simulink model "Microgrid_ITM_client"  (R2025b)
settings: Solver=FixedStepAuto  StartTime=0.0  StopTime=0.05  FixedStep=5e-7  RelTol=1e-3
InitFcn:
  | clear;
  | setup_two_pc_cosim();
  | clear Server_co_TLM Client_co_TLM
  | rehash;
  | release_two_pc_tcp_ports();
  | Vline = 380;%Rated RMS of Line Voltage
  | Vdc = 750;%DC voltage
  | Vac = sqrt(2)*Vline/sqrt(3);%Amplitude of Phase to Neutral Volatge
  | P = 10*10^(3);%Rate Power
  | f=50;%Rated Frequency
  | Wb=2*pi*f;%Rated Angular Frequency
  | fsw1=10e3;  %INV1 switching frequency
  | 
  | %Base Value of PU System
  | Vp=Vac;%Voltage
  | Ip=2/3*P/Vp;%Current
  | Zb = Vp/Ip;%Impedance
  | Lb=Zb/2/pi/f;%Inductance
  | Cb=1/(2*pi*f*Zb);%Capacitance
  | 
  | %Network Parameters
  | R1_pu=0.1/Zb;R1=R1_pu*Zb;
  | R2_pu=0.1/Zb;R2=R2_pu*Zb;
  | R3_pu=0.1/Zb;R3=R3_pu*Zb;
  | R4_pu=0.1/Zb;R4=R4_pu*Zb;
  | L1_pu=2e-3/Lb;L1=L1_pu*Lb;
  | L2_pu=2e-3/Lb;L2=L2_pu*Lb;
  | L3_pu=2e-3/Lb;L3=L3_pu*Lb;
  | L4_pu=2e-3/Lb;L4=L4_pu*Lb;
  | 
  | %Load Parameters
  | Rload1_pu=Vp/Ip/Zb;Rload1=Rload1_pu*Zb;
  | Rload2_pu=Vp/Ip/Zb;Rload2=Rload2_pu*Zb;
  | Rload3_pu=Vp/Ip/Zb;Rload3=Rload3_pu*Zb;
  | 
  | %Virtual Impedance
  | Rv_pu=0.05;
  | Xv_pu=0.2;
  | 
  | Lc=2.5e-3;
StopFcn:
  | %% StopFcn: save ITM client-side results
  | 
  | % 获取模型所在目录
  | modelName = bdroot;
  | modelFile = get_param(modelName, 'FileName');
  | 
  | if isempty(modelFile)
  |     % 模型还没有保存时，使用当前工作目录
  |     modelDir = pwd;
  | else
  |     modelDir = fileparts(modelFile);
  | end
  | 
  | % 定义并创建 result 文件夹
  | resultDir = fullfile(modelDir, 'result');
  | 
  | if ~exist(resultDir, 'dir')
  |     mkdir(resultDir);
  | end
  | 
  | % 需要保存的 Client-side 工作区变量
  | variableNames = {
  |     'client_voltage'
  |     'client_current'
  |     'client_PQ'
  |     'client_omega'
  | };
  | 
  | clientITMData = struct();
  | 
  | for k = 1:numel(variableNames)
  | 
  |     originalName = variableNames{k};
  |     saveName = [originalName, '_client_ITM'];
  | 
  |     variableExists = evalin( ...
  |         'base', ...
  |         sprintf('exist(''%s'', ''var'')', originalName));
  | 
  |     if variableExists
  |         clientITMData.(saveName) = evalin('base', originalName);
  |     else
  |         warning( ...
  |             'StopFcn:MissingVariable', ...
  |             'Variable "%s" was not found in the base workspace.', ...
  |             originalName);
  |     end
  | end
  | 
  | % 保存文件
  | saveFile = fullfile(resultDir, 'client_ITM.mat');
  | save(saveFile, '-struct', 'clientITMData');
  | 
  | fprintf('ITM client-side results saved to:\n%s\n', saveFile);
undefined symbols (not defined in the file or in its folder): DiscIntNeverNeededParam
libraries: spsThreePhaseSeriesRLCBranchLib x4, spsControlledCurrentSourceLib x3, spsControlledVoltageSourceLib x3, slpidlib x3, spsabctodq0Lib x3, spsThreePhaseVIMeasurementLib x3, spsThreePhaseTransformerTwoWindingsLib x2, spsDCVoltageSourceLib x1, spsGroundLib x1, spsPWMGenerator2LevelLib x1, spsPower3phInstantaneousLib x1, spsdq0toabcLib x1
settings Model: Creator=L  LastModifiedBy=Yuming
settings SolverCC: AlgebraicLoopSolver=TrustRegion
settings DataIOCC: LimitDataPoints=on  SaveFormat=Array  ReturnWorkspaceOutputs=off
settings OptimizationCC: ReuseModelBlockBuffer=off  LifeSpan=inf
settings DebuggingCC: UnderspecifiedInitializationDetection=Classic  MergeDetectMultiDrivingBlocksExec=none  SolverPrmCheckMsg=warning  UnconnectedInputMsg=warning  UnconnectedOutputMsg=warning  UnconnectedLineMsg=warning  StateNameClashWarn=warning  SFUnexpectedBacktrackingDiag=warning  SFNoUnconditionalDefaultTransitionDiag=warning  SFExecutionAtInitializationDiag=none  ArithmeticOperatorsInVariantConditions=warning
settings HardwareCC: ProdBitPerPointer=32.0  ProdBitPerSizeT=32.0  ProdBitPerPtrDiffT=32.0  ProdLargestAtomicFloat=None  ProdIntDivRoundTo=Undefined  ProdEndianess=Unspecified  ProdWordSize=32.0  ProdHWDeviceType=32-bit Generic
settings ModelReferenceCC: EnableRefExpFcnMdlSchedulingChecks=on  PropagateSignalLabelsOutOfModel=off
settings SFSimCC: SimUseLocalCustomCode=off  CustomCodeUndefinedFunction=UseInterfaceOnly
settings RTWCC: RTWUseLocalCustomCode=off  GPUComputeCapability=3.5  DLArmComputeVersion=19.05
settings CodeAppCC: StateflowObjectComments=on
settings GRTTargetCC: TargetLangStandard=C89/C90 (ANSI)
settings ConfigComp: CovMetricSettings=dw  CovSaveCumulativeToWorkspaceVar=on  CovSaveSingleToWorkspaceVar=on  CovExternalEMLEnable=off
settings SimscapeCC: SimscapeNormalizeSystem=off

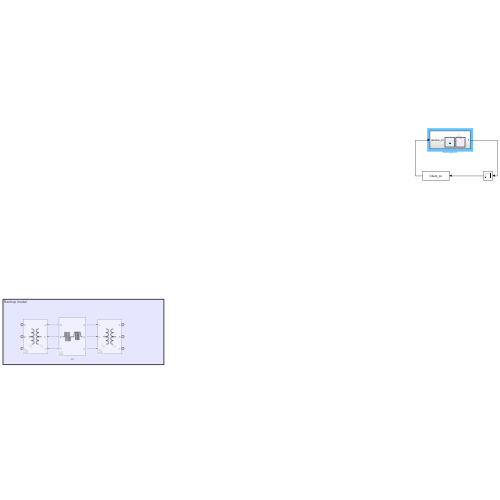
[thumbnail: Simulink's stored preview of the top-level diagram]
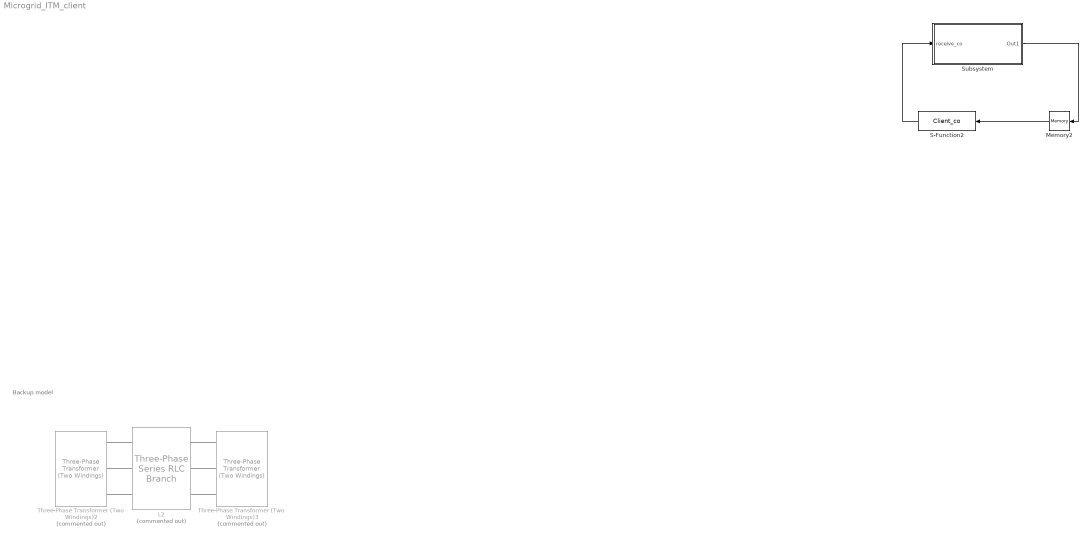
== system Microgrid_ITM_client ==
  note: Backup model
  L2 : spsThreePhaseSeriesRLCBranchLib/Three-Phase Series RLC Branch  Commented=on  LConnTagsString=A|B|C  RConnTagsString=A|B|C  BranchType=RL  Resistance=R2  Inductance=L2  Capacitance=1e-6  Measurements=None
  Memory2 : Memory
  S-Function2 : S-Function  FunctionName=Client_co  SFunctionDeploymentMode=off  EnableBusSupport=off
  Subsystem : Subsystem
  Three-Phase Transformer (Two Windings)2 : spsThreePhaseTransformerTwoWindingsLib/Three-Phase Transformer (Two Windings)  Commented=on  Winding1Connection=Yg  Winding2Connection=Yg  CoreType=Three single-phase transformers  SetSaturation=off  Hysteresis=off  DataFile='hysteresis'  SetInitialFlux=off  Measurements=None  UNITS=pu  NominalPower=[ 250e6 , 50 ]  Winding1=[ 380e3 , 0.002 , 0.08 ]  Winding2=[ 33e3 , 0.002 , 0.08 ]  Rm=500  Lm=500  L0=0.5  Saturation=[ 0,0 ; 0.0024,1.2 ; 1.0,1.52 ]  InitialFluxes=[ 0.8 , -0.8 , 0.7 ]  BreakLoop=off  DiscreteSolver=Trapezoidal iterative  DataType=off  TransfoNumber=1
  Three-Phase Transformer (Two Windings)3 : spsThreePhaseTransformerTwoWindingsLib/Three-Phase Transformer (Two Windings)  Commented=on  Winding1Connection=Yg  Winding2Connection=Yg  CoreType=Three single-phase transformers  SetSaturation=off  Hysteresis=off  DataFile='hysteresis'  SetInitialFlux=off  Measurements=None  UNITS=pu  NominalPower=[ 250e6 , 50 ]  Winding1=[ 33e3 , 0.002 , 0.08 ]  Winding2=[ 380 , 0.002 , 0.08 ]  Rm=500  Lm=500  L0=0.5  Saturation=[ 0,0 ; 0.0024,1.2 ; 1.0,1.52 ]  InitialFluxes=[ 0.8 , -0.8 , 0.7 ]  BreakLoop=off  DiscreteSolver=Trapezoidal iterative  DataType=off  TransfoNumber=1
  wires:
  Memory2/1 -> S-Function2/1
  S-Function2/1 -> Subsystem/1(receive_co)
  Subsystem/1(Out1) -> Memory2/1
  connections:
  Three-Phase Transformer (Two Windings)3/RConn1 -- L2/RConn1
  Three-Phase Transformer (Two Windings)3/RConn2 -- L2/RConn2
  Three-Phase Transformer (Two Windings)3/RConn3 -- L2/RConn3
  Three-Phase Transformer (Two Windings)2/RConn1 -- L2/LConn1
  Three-Phase Transformer (Two Windings)2/RConn2 -- L2/LConn2
  Three-Phase Transformer (Two Windings)2/RConn3 -- L2/LConn3

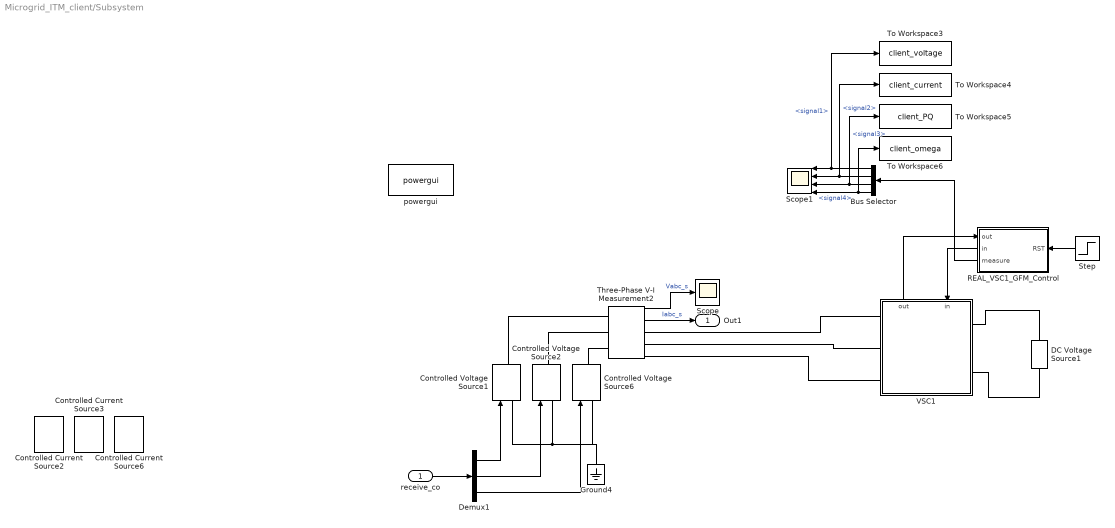
== system Microgrid_ITM_client/Subsystem ==
  receive_co : Inport
  Bus Selector : BusSelector  OutputSignals=signal1,signal2,signal3,signal4
  Controlled Current Source2 : spsControlledCurrentSourceLib/Controlled Current Source  Initialize=on  Source_Type=AC  Amplitude=0  Phase=0  Frequency=0  Measurements=None
  Controlled Current Source3 : spsControlledCurrentSourceLib/Controlled Current Source  Initialize=on  Source_Type=AC  Amplitude=0  Phase=0  Frequency=0  Measurements=None
  Controlled Current Source6 : spsControlledCurrentSourceLib/Controlled Current Source  Initialize=on  Source_Type=AC  Amplitude=0  Phase=0  Frequency=0  Measurements=None
  Controlled Voltage Source1 : spsControlledVoltageSourceLib/Controlled Voltage Source  Initialize=on  Source_Type=AC  Amplitude=0  Phase=0  Frequency=0  Measurements=None
  Controlled Voltage Source2 : spsControlledVoltageSourceLib/Controlled Voltage Source  Initialize=on  Source_Type=AC  Amplitude=0  Phase=0  Frequency=0  Measurements=None
  Controlled Voltage Source6 : spsControlledVoltageSourceLib/Controlled Voltage Source  Initialize=on  Source_Type=AC  Amplitude=0  Phase=0  Frequency=0  Measurements=None
  DC Voltage Source1 : spsDCVoltageSourceLib/DC Voltage Source  Amplitude=Vdc  Measurements=None
  Demux1 : Demux  Outputs=3
  Ground4 : spsGroundLib/Ground  LConnTagsString=a
  REAL_VSC1_GFM_Control : Subsystem
      settings: PortSchema="{\"entries\":[{\"content\":{\"sides\":[{\"content\":{\"connectorIds\":[\"In1\"]},\"type\":\"ConnectorPlacement.EquallySpacedRectSide\",\"uuid\":\"8a24280a-bafa-4af5-a0f6-406aa9a59b4a\"},{\"content\":{\"connectorIds\":[\"In2\",\"Out1\",\"Out2\"],\"side\":\"RIGHT\"},\"type\":\"ConnectorPlacement.EquallySpacedRectSide\",\"uuid\":\"7d4db3bb-9035-4630-ac97-c56e5fe5f777\"},{\"content\":{\"side\":\"TOP\"},\"type\":\"ConnectorPlacement.EquallySpacedRectSide\",\"uuid\":\"cf83f05c-de7f-4d84-9d8a-6900bb43b99f\"}]},\"type\":\"ConnectorPlacement.EquallySpacedConnector\",\"uuid\":\"3f42a8c1-e25b-4642-96cc-07219abe8890\"}],\"packageUris\":[\"http://schema.mathworks.com/mf0/Connector/R2020b\"],\"version\":\"1.0\"}"
  Scope : Scope
      settings: ActiveDisplayYMinimum=-5.8273159155410254E+163  ActiveDisplayYMaximum=5.8951340842267878E+163  DataLoggingVariableName=ScopeData5
  Scope1 : Scope  NumInputPorts=4
      settings: ActiveDisplayYMinimum=-417.44619371330521  ActiveDisplayYMaximum=395.41957020213545  DataLoggingVariableName=ScopeData4
  Step : Step  Time=0.2  SampleTime=0
  Three-Phase V-I Measurement2 : spsThreePhaseVIMeasurementLib/Three-Phase V-I Measurement  VoltageMeasurement=phase-to-ground  SetLabelV=off  LabelV=Vabc_s  Vpu=off  VpuLL=off  CurrentMeasurement=yes  SetLabelI=off  LabelI=Iabc_s  Ipu=off  Pbase=100e6  Vbase=500e3  OutputType=Complex  PhasorSimulation=off  PSBequivalent=0
  To Workspace3 : ToWorkspace  VariableName=client_voltage  SaveFormat=Timeseries  SampleTime=-1
  To Workspace4 : ToWorkspace  VariableName=client_current  SaveFormat=Timeseries  SampleTime=-1
  To Workspace5 : ToWorkspace  VariableName=client_PQ  SaveFormat=Timeseries  SampleTime=-1
  To Workspace6 : ToWorkspace  VariableName=client_omega  SaveFormat=Timeseries  SampleTime=-1
  VSC1 : Subsystem
      settings: PortSchema="{\"entries\":[{\"content\":{\"sides\":[{\"content\":{\"connectorIds\":[\"LConn1\",\"LConn2\"]},\"type\":\"ConnectorPlacement.EquallySpacedRectSide\",\"uuid\":\"f9a47b7a-7ab9-4bc4-ba6a-b9374cb03391\"},{\"content\":{\"connectorIds\":[\"RConn1\",\"RConn2\",\"RConn3\"],\"side\":\"RIGHT\"},\"type\":\"ConnectorPlacement.EquallySpacedRectSide\",\"uuid\":\"cfb0475f-9637-449c-a598-06e77c9a1f18\"},{\"content\":{\"connectorIds\":[\"In1\",\"Out1\"],\"side\":\"TOP\"},\"type\":\"ConnectorPlacement.EquallySpacedRectSide\",\"uuid\":\"93622264-4e82-4ec9-8ad8-ec19c934a5ef\"},{\"content\":{\"side\":\"HIDDEN\"},\"type\":\"ConnectorPlacement.EquallySpacedRectSide\",\"uuid\":\"56686535-bc45-40fb-9bd4-cc49f520b447\"}]},\"type\":\"ConnectorPlacement.EquallySpacedConnector\",\"uuid\":\"6064451f-78f0-465c-b58b-22fa19e3979e\"}],\"packageUris\":[\"http://schema.mathworks.com/mf0/Connector/R2020b\"],\"version\":\"1.0\"}"
  powergui : spspowerguiLib/powergui  Priority=1  SimulationMode=Discrete  SampleTime=5e-7  frequency=60  Iterations=50  frequencyindice=0  Pbase=100e6  ErrMax=1e-4  UnitsV=kV  UnitsW=MW  buscounter=0  FunctionMessages=off  echomessages=off  EnableUseOfTLC=off  CurrentSourceSwitches=off  DisableSnubberDevices=off  DisableRonSwitches=off  DisableVfSwitches=off  DisplayEquations=off  AutomaticDiscreteSolvers=off  SolverType=Tustin/Backward Euler (TBE)  Interpol=off  ExternalGateDelay=off  methode=off  Ts=100  x0status=blocks  SPID=on  SwTol=0  HookPort=off  NonlinearTolerance=1e-4  nMaxIteration=100  ContinueOnMaxIteration=off  RestoreLinks=warning  ResistiveCurrentMeasurement=off  Frange=[0:2:500]  Ylog=off  Xlog=on  ShowGrid=off  save=off  variable=ZData  structure=0  ZoomFFT=off  StartTime=0.0  cycles=1  DisplayStyle=1  fundamental=60  FreqAxis=off  MaxFrequency=1000  frequencyindicesteady=1  RmsSteady=1  display=off
  Out1 : Outport
  wires:
  VSC1/1(out) -> REAL_VSC1_GFM_Control/2(out)
  Step/1 -> REAL_VSC1_GFM_Control/1(RST)
  REAL_VSC1_GFM_Control/1(in) -> VSC1/1(in)
  Demux1/2 -> Controlled Voltage Source2/1
  Demux1/3 -> Controlled Voltage Source6/1
  receive_co/1 -> Demux1/1
  Demux1/1 -> Controlled Voltage Source1/1
  REAL_VSC1_GFM_Control/2(measure) -> Bus Selector/1
  Bus Selector/1 -> To Workspace3/1, Scope1/1  "<signal1>"
  Bus Selector/3 -> To Workspace5/1, Scope1/3  "<signal3>"
  Bus Selector/4 -> To Workspace6/1, Scope1/4  "<signal4>"
  Bus Selector/2 -> To Workspace4/1, Scope1/2  "<signal2>"
  Three-Phase V-I Measurement2/1 -> Scope/1  "Vabc_s"
  Three-Phase V-I Measurement2/2 -> Out1/1  "Iabc_s"
  connections:
  DC Voltage Source1/RConn1 -- VSC1/LConn1
  VSC1/LConn2 -- DC Voltage Source1/LConn1
  Controlled Voltage Source1/RConn1 -- Three-Phase V-I Measurement2/LConn1
  Ground4/LConn1 -- Controlled Voltage Source6/LConn1 -- Controlled Voltage Source1/LConn1 -- Controlled Voltage Source2/LConn1
  Controlled Voltage Source2/RConn1 -- Three-Phase V-I Measurement2/LConn2
  Controlled Voltage Source6/RConn1 -- Three-Phase V-I Measurement2/LConn3
  Three-Phase V-I Measurement2/RConn1 -- VSC1/RConn1
  Three-Phase V-I Measurement2/RConn2 -- VSC1/RConn2
  Three-Phase V-I Measurement2/RConn3 -- VSC1/RConn3

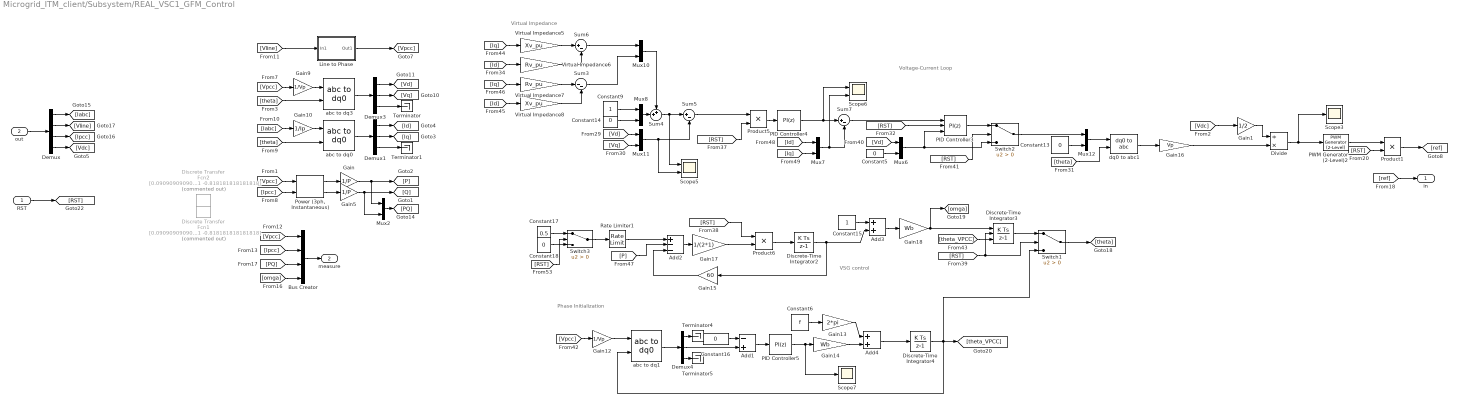
== system Microgrid_ITM_client/Subsystem/REAL_VSC1_GFM_Control ==
  note: Voltage-Current Loop
  note: VSG control
  note: Virtual Impedance
  note: Phase Initialization
  RST : Inport
  out : Inport  Port=2
  Add1 : Sum  Inputs=-+
  Add2 : Sum  Inputs=+--
  Add3 : Sum
  Add4 : Sum
  Bus Creator : BusCreator  Inputs=4
  Constant{5,13..14,16} (4 alike) : Constant  Value=0
  Constant15 : Constant
  Constant17 : Constant  Value=0.5  SampleTime=-1
  Constant18 : Constant  Value=0  SampleTime=-1
  Constant6 : Constant  Value=f
  Constant9 : Constant  SampleTime=-1
  Demux : Demux
  Demux1 : Demux  Outputs=3
  Demux3 : Demux  Outputs=3
  Demux4 : Demux  Outputs=3
  Discrete Transfer Fcn1 : DiscreteTransferFcn  Commented=on  Numerator=[0.090909090909091 0.090909090909091]  Denominator=[1 -0.818181818181818]
  Discrete Transfer Fcn2 : DiscreteTransferFcn  Commented=on  Numerator=[0.090909090909091 0.090909090909091]  Denominator=[1 -0.818181818181818]
  Discrete-Time Integrator2 : DiscreteIntegrator  SampleTime=1/fsw1  ICPrevOutput=DiscIntNeverNeededParam  ICPrevScaledInput=DiscIntNeverNeededParam
  Discrete-Time Integrator3 : DiscreteIntegrator  ExternalReset=rising  InitialConditionSource=external  SampleTime=1/fsw1  ICPrevOutput=DiscIntNeverNeededParam  ICPrevScaledInput=DiscIntNeverNeededParam
  Discrete-Time Integrator4 : DiscreteIntegrator  SampleTime=1/fsw1  ICPrevOutput=DiscIntNeverNeededParam  ICPrevScaledInput=DiscIntNeverNeededParam
  Divide : Product  Inputs=/*
  Gain : Gain  Gain=1/P
  Gain1 : Gain  Gain=1/2
  Gain10 : Gain  Gain=1/Ip
  Gain12 : Gain  Gain=1/Vp
  Gain13 : Gain  Gain=2*pi
  Gain14 : Gain  Gain=Wb
  Gain15 : Gain  Gain=60
  Gain16 : Gain  Gain=Vp
  Gain17 : Gain  Gain=1/(2*1)
  Gain18 : Gain  Gain=Wb
  Gain5 : Gain  Gain=1/P
  Gain9 : Gain  Gain=1/Vp
  Line to Phase : Subsystem
  Mux{2,6..8,10..12} (7 alike) : Mux  Inputs=2
  PID Controller3 : slpidlib/PID Controller  Controller=PI  Form=Parallel  TimeDomain=Discrete-time  UseExternalTs=off  SampleTime=1/fsw1  IntegratorMethod=Forward Euler  FilterMethod=Forward Euler  ControllerParametersSource=internal  P=0.5  I=100  UseKiTs=off  D=0  UseExternalDerivativeSource=off  N=100  UseFilter=on  TunerSelectOption=Transfer Function Based (PID Tuner App)  InitialConditionSource=external  InitialConditionForIntegrator=0  InitialConditionForFilter=0  DifferentiatorICPrevScaledInput=0  ExternalReset=rising  TrackingMode=off  Kt=1  LimitOutput=off  SatLimitsSource=internal  UpperSaturationLimit=inf  LowerSaturationLimit=-inf  LinearizeAsGain=on  AntiWindupMode=none  Kb=1  LimitIntegrator=off  UpperIntegratorSaturationLimit=inf  LowerIntegratorSaturationLimit=-inf  POutMin=[]  POutMax=[]  IOutMin=[]  IOutMax=[]  DOutMin=[]  DOutMax=[]  NOutMin=[]  NOutMax=[]  SumOutMin=[]  SumOutMax=[]  SaturationOutMin=[]  SaturationOutMax=[]  PParamMin=[]  PParamMax=[]  IParamMin=[]  IParamMax=[]  DParamMin=[]  DParamMax=[]  NParamMin=[]  NParamMax=[]  KbParamMin=[]  KbParamMax=[]  KtParamMin=[]  KtParamMax=[]  KbOutMin=[]  KbOutMax=[]  KtOutMin=[]  KtOutMax=[]  IntegratorOutMin=[]  IntegratorOutMax=[]  FilterOutMin=[]  FilterOutMax=[]  SumI1OutMin=[]  SumI1OutMax=[]  SumI2OutMin=[]  SumI2OutMax=[]  SumI3OutMin=[]  SumI3OutMax=[]  SumI4OutMin=[]  SumI4OutMax=[]  SumDOutMin=[]  SumDOutMax=[]  DifferentiatorOutMin=[]  DifferentiatorOutMax=[]  FilterDiffOutCoefMin=[]  FilterDiffOutCoefMax=[]  ReciprocalOutMin=[]  ReciprocalOutMax=[]  SumDenOutMin=[]  SumDenOutMax=[]  SumNumOutMin=[]  SumNumOutMax=[]  DivideOutMin=[]  DivideOutMax=[]  UdiffTsProdOutMin=[]  UdiffTsProdOutMax=[]  NTsProdOutMin=[]  NTsProdOutMax=[]  UintegralTsProdOutMin=[]  UintegralTsProdOutMax=[]  UngainTsProdOutMin=[]  UngainTsProdOutMax=[]  ClampingZeroOutDataTypeStr=Inherit: Inherit via back propagation  ClampingZeroOutMin=[]  ClampingZeroOutMax=[]  FilterDenConstantOutDataTypeStr=Inherit: Inherit via back propagation  FilterDenConstantOutMin=[]  FilterDenConstantOutMax=[]  PCopyOutDataTypeStr=Inherit: Inherit via back propagation  PCopyOutMin=[]  PCopyOutMax=[]  NCopyOutDataTypeStr=Inherit: Inherit via back propagation  NCopyOutMin=[]  NCopyOutMax=[]  IntegratorContinuousStateAttributes=''  IntegratorStateMustResolveToSignalObject=off  IntegratorRTWStateStorageClass=Auto  FilterContinuousStateAttributes=''  FilterStateMustResolveToSignalObject=off  FilterRTWStateStorageClass=Auto  ParallelPVariant=InternalParameters  IdealPVariant=Disabled  IVariant=InternalParameters  DVariant=Disabled  IntegratorVariant=Discrete  SatVariant=Disabled  AWVariant=Passthrough  PCopyVariant=Disabled  TRVariant=Disabled  FdbkBlocksVariant=Forward  IdealPFdbkVariant=Disabled  SatFdbkVariant=Disabled  DerivativeFilterVariant=Disabled  NVariant=Disabled  NCopyVariant=Disabled_SignalSpec  FilterICVariant=Disabled  IntegratorICVariant=ExternalICs  ExternalResetVariant=ExternalReset  TRSumVariant=Passthrough  SumFdbkVariant=Disabled  SumVariant=Sum_PI  TsampFilterVariant=InternalTs  TsampNgainVariant=Passthrough  TsampIntegralVariant=Disabled_SignalSpec  ExternalSaturationOutDataTypeStr=Inherit: Same as second input  DerivativeSourceVariant=Disabled  PreIntVariant=InternalPreInt
  PID Controller4 : slpidlib/PID Controller  Controller=PI  Form=Parallel  TimeDomain=Discrete-time  UseExternalTs=off  SampleTime=1/fsw1  IntegratorMethod=Forward Euler  FilterMethod=Forward Euler  ControllerParametersSource=internal  P=0.1  I=200  UseKiTs=off  D=0  UseExternalDerivativeSource=off  N=100  UseFilter=on  TunerSelectOption=Transfer Function Based (PID Tuner App)  InitialConditionSource=internal  InitialConditionForIntegrator=0  InitialConditionForFilter=0  DifferentiatorICPrevScaledInput=0  ExternalReset=none  TrackingMode=off  Kt=1  LimitOutput=off  SatLimitsSource=internal  UpperSaturationLimit=inf  LowerSaturationLimit=-inf  LinearizeAsGain=on  AntiWindupMode=none  Kb=1  LimitIntegrator=off  UpperIntegratorSaturationLimit=inf  LowerIntegratorSaturationLimit=-inf  POutMin=[]  POutMax=[]  IOutMin=[]  IOutMax=[]  DOutMin=[]  DOutMax=[]  NOutMin=[]  NOutMax=[]  SumOutMin=[]  SumOutMax=[]  SaturationOutMin=[]  SaturationOutMax=[]  PParamMin=[]  PParamMax=[]  IParamMin=[]  IParamMax=[]  DParamMin=[]  DParamMax=[]  NParamMin=[]  NParamMax=[]  KbParamMin=[]  KbParamMax=[]  KtParamMin=[]  KtParamMax=[]  KbOutMin=[]  KbOutMax=[]  KtOutMin=[]  KtOutMax=[]  IntegratorOutMin=[]  IntegratorOutMax=[]  FilterOutMin=[]  FilterOutMax=[]  SumI1OutMin=[]  SumI1OutMax=[]  SumI2OutMin=[]  SumI2OutMax=[]  SumI3OutMin=[]  SumI3OutMax=[]  SumI4OutMin=[]  SumI4OutMax=[]  SumDOutMin=[]  SumDOutMax=[]  DifferentiatorOutMin=[]  DifferentiatorOutMax=[]  FilterDiffOutCoefMin=[]  FilterDiffOutCoefMax=[]  ReciprocalOutMin=[]  ReciprocalOutMax=[]  SumDenOutMin=[]  SumDenOutMax=[]  SumNumOutMin=[]  SumNumOutMax=[]  DivideOutMin=[]  DivideOutMax=[]  UdiffTsProdOutMin=[]  UdiffTsProdOutMax=[]  NTsProdOutMin=[]  NTsProdOutMax=[]  UintegralTsProdOutMin=[]  UintegralTsProdOutMax=[]  UngainTsProdOutMin=[]  UngainTsProdOutMax=[]  ClampingZeroOutDataTypeStr=Inherit: Inherit via back propagation  ClampingZeroOutMin=[]  ClampingZeroOutMax=[]  FilterDenConstantOutDataTypeStr=Inherit: Inherit via back propagation  FilterDenConstantOutMin=[]  FilterDenConstantOutMax=[]  PCopyOutDataTypeStr=Inherit: Inherit via back propagation  PCopyOutMin=[]  PCopyOutMax=[]  NCopyOutDataTypeStr=Inherit: Inherit via back propagation  NCopyOutMin=[]  NCopyOutMax=[]  IntegratorContinuousStateAttributes=''  IntegratorStateMustResolveToSignalObject=off  IntegratorRTWStateStorageClass=Auto  FilterContinuousStateAttributes=''  FilterStateMustResolveToSignalObject=off  FilterRTWStateStorageClass=Auto  ParallelPVariant=InternalParameters  IdealPVariant=Disabled  IVariant=InternalParameters  DVariant=Disabled  IntegratorVariant=Discrete  SatVariant=Disabled  AWVariant=Passthrough  PCopyVariant=Disabled  TRVariant=Disabled  FdbkBlocksVariant=Forward  IdealPFdbkVariant=Disabled  SatFdbkVariant=Disabled  DerivativeFilterVariant=Disabled  NVariant=Disabled  NCopyVariant=Disabled_SignalSpec  FilterICVariant=Disabled  IntegratorICVariant=InternalICs  ExternalResetVariant=Disabled  TRSumVariant=Passthrough  SumFdbkVariant=Disabled  SumVariant=Sum_PI  TsampFilterVariant=InternalTs  TsampNgainVariant=Passthrough  TsampIntegralVariant=Disabled_SignalSpec  ExternalSaturationOutDataTypeStr=Inherit: Same as second input  DerivativeSourceVariant=Disabled  PreIntVariant=InternalPreInt
  PID Controller5 : slpidlib/PID Controller  Controller=PI  Form=Parallel  TimeDomain=Discrete-time  UseExternalTs=off  SampleTime=1/fsw1  IntegratorMethod=Forward Euler  FilterMethod=Forward Euler  ControllerParametersSource=internal  P=2  I=5  UseKiTs=off  D=0  UseExternalDerivativeSource=off  N=100  UseFilter=on  TunerSelectOption=Transfer Function Based (PID Tuner App)  InitialConditionSource=internal  InitialConditionForIntegrator=0  InitialConditionForFilter=0  DifferentiatorICPrevScaledInput=0  ExternalReset=none  TrackingMode=off  Kt=1  LimitOutput=off  SatLimitsSource=internal  UpperSaturationLimit=inf  LowerSaturationLimit=-inf  LinearizeAsGain=on  AntiWindupMode=none  Kb=1  LimitIntegrator=off  UpperIntegratorSaturationLimit=inf  LowerIntegratorSaturationLimit=-inf  POutMin=[]  POutMax=[]  IOutMin=[]  IOutMax=[]  DOutMin=[]  DOutMax=[]  NOutMin=[]  NOutMax=[]  SumOutMin=[]  SumOutMax=[]  SaturationOutMin=[]  SaturationOutMax=[]  PParamMin=[]  PParamMax=[]  IParamMin=[]  IParamMax=[]  DParamMin=[]  DParamMax=[]  NParamMin=[]  NParamMax=[]  KbParamMin=[]  KbParamMax=[]  KtParamMin=[]  KtParamMax=[]  KbOutMin=[]  KbOutMax=[]  KtOutMin=[]  KtOutMax=[]  IntegratorOutMin=[]  IntegratorOutMax=[]  FilterOutMin=[]  FilterOutMax=[]  SumI1OutMin=[]  SumI1OutMax=[]  SumI2OutMin=[]  SumI2OutMax=[]  SumI3OutMin=[]  SumI3OutMax=[]  SumI4OutMin=[]  SumI4OutMax=[]  SumDOutMin=[]  SumDOutMax=[]  DifferentiatorOutMin=[]  DifferentiatorOutMax=[]  FilterDiffOutCoefMin=[]  FilterDiffOutCoefMax=[]  ReciprocalOutMin=[]  ReciprocalOutMax=[]  SumDenOutMin=[]  SumDenOutMax=[]  SumNumOutMin=[]  SumNumOutMax=[]  DivideOutMin=[]  DivideOutMax=[]  UdiffTsProdOutMin=[]  UdiffTsProdOutMax=[]  NTsProdOutMin=[]  NTsProdOutMax=[]  UintegralTsProdOutMin=[]  UintegralTsProdOutMax=[]  UngainTsProdOutMin=[]  UngainTsProdOutMax=[]  ClampingZeroOutDataTypeStr=Inherit: Inherit via back propagation  ClampingZeroOutMin=[]  ClampingZeroOutMax=[]  FilterDenConstantOutDataTypeStr=Inherit: Inherit via back propagation  FilterDenConstantOutMin=[]  FilterDenConstantOutMax=[]  PCopyOutDataTypeStr=Inherit: Inherit via back propagation  PCopyOutMin=[]  PCopyOutMax=[]  NCopyOutDataTypeStr=Inherit: Inherit via back propagation  NCopyOutMin=[]  NCopyOutMax=[]  IntegratorContinuousStateAttributes=''  IntegratorStateMustResolveToSignalObject=off  IntegratorRTWStateStorageClass=Auto  FilterContinuousStateAttributes=''  FilterStateMustResolveToSignalObject=off  FilterRTWStateStorageClass=Auto  ParallelPVariant=InternalParameters  IdealPVariant=Disabled  IVariant=InternalParameters  DVariant=Disabled  IntegratorVariant=Discrete  SatVariant=Disabled  AWVariant=Passthrough  PCopyVariant=Disabled  TRVariant=Disabled  FdbkBlocksVariant=Forward  IdealPFdbkVariant=Disabled  SatFdbkVariant=Disabled  DerivativeFilterVariant=Disabled  NVariant=Disabled  NCopyVariant=Disabled_SignalSpec  FilterICVariant=Disabled  IntegratorICVariant=InternalICs  ExternalResetVariant=Disabled  TRSumVariant=Passthrough  SumFdbkVariant=Disabled  SumVariant=Sum_PI  TsampFilterVariant=InternalTs  TsampNgainVariant=Passthrough  TsampIntegralVariant=Disabled_SignalSpec  ExternalSaturationOutDataTypeStr=Inherit: Same as second input  DerivativeSourceVariant=Disabled  PreIntVariant=InternalPreInt
  PWM Generator (2-Level)2 : spsPWMGenerator2LevelLib/PWM Generator (2-Level)  ModulatorType=Three-phase bridge (6 pulses)  ModulatorMode=Unsynchronized  Fc=fsw1  Pc=0  nF=27  MinMax="[ -1  1 ]"  SamplingTechnique=Asymmetrical regular (double edge)  ModulatingSignals=off  m=0.8  Freq=60  Phase=0  Ts=0  ShowCarrierOutport=off
  "Power (3ph, Instantaneous)" : spsPower3phInstantaneousLib/Power (3ph, Instantaneous)
  Product1 : Product
  Product5 : Product
  Product6 : Product
  Rate Limiter1 : RateLimiter  RisingSlewLimit=5  FallingSlewLimit=-5  SampleTimeMode=inherited
  Scope3 : Scope
      settings: ActiveDisplayYMinimum=-3.23588  ActiveDisplayYMaximum=3.22923
  Scope5 : Scope  NumInputPorts=2
      settings: ActiveDisplayYMinimum=-0.89875  ActiveDisplayYMaximum=1.61871
  Scope6 : Scope  NumInputPorts=2
      settings: ActiveDisplayYMinimum=-0.00056  ActiveDisplayYMaximum=0.00032  DataLoggingVariableName=ScopeData2
  Scope7 : Scope
      settings: ActiveDisplayYMinimum=-0.17841  ActiveDisplayYMaximum=0.07598  DataLoggingVariableName=ScopeData3
  Sum3 : Sum  Inputs=|--
  Sum4 : Sum  Inputs=++|
  Sum5 : Sum  Inputs=|+-
  Sum6 : Sum  Inputs=|+-
  Sum7 : Sum  Inputs=|+-
  Switch1 : Switch  Criteria=u2 > Threshold  SaturateOnIntegerOverflow=off  InputSameDT=off
  Switch2 : Switch  Criteria=u2 > Threshold  SaturateOnIntegerOverflow=off  InputSameDT=off
  Switch3 : Switch  Criteria=u2 > Threshold  SaturateOnIntegerOverflow=off  InputSameDT=off
  Terminator{,1,4..5} (4 alike) : Terminator
  Virtual Impedance5 : Gain  Gain=Xv_pu
  Virtual Impedance6 : Gain  Gain=Rv_pu
  Virtual Impedance7 : Gain  Gain=Rv_pu
  Virtual Impedance8 : Gain  Gain=Xv_pu
  abc to dq0 : spsabctodq0Lib/abc to dq0  Alignment=90 degrees behind phase A axis
  abc to dq1 : spsabctodq0Lib/abc to dq0  Alignment=90 degrees behind phase A axis
  abc to dq3 : spsabctodq0Lib/abc to dq0  Alignment=90 degrees behind phase A axis
  dq0 to abc1 : spsdq0toabcLib/dq0 to abc  Alignment=90 degrees behind phase A axis
  in : Outport
  measure : Outport  Port=2
  wires:
  [RST] -> Product1/2
  Gain16/1 -> Divide/2
  PWM Generator (2-Level)2/1 -> Product1/1
  Product1/1 -> [ref]
  Gain1/1 -> Divide/1
  Divide/1 -> PWM Generator (2-Level)2/1, Scope3/1
  [Vdc] -> Gain1/1
  [ref] -> in/1
  Gain5/1 -> [Q], Mux2/2
  Gain/1 -> [P], Mux2/1
  Line to Phase/1(Out1) -> [Vpcc]
  [Vline] -> Line to Phase/1(In1)
  Demux1/2 -> [Iq]
  Demux1/3 -> Terminator1/1
  Demux1/1 -> [Id]
  abc to dq0/1 -> Demux1/1
  [Iabc] -> Gain10/1
  Gain9/1 -> abc to dq3/1
  abc to dq3/1 -> Demux3/1
  Gain10/1 -> abc to dq0/1
  Demux3/1 -> [Vd]
  [theta] -> abc to dq0/2
  [theta] -> abc to dq3/2
  Demux3/3 -> Terminator/1
  [Vpcc] -> Gain9/1
  Demux3/2 -> [Vq]
  [Vpcc] -> "Power (3ph, Instantaneous)"/1
  [Ipcc] -> "Power (3ph, Instantaneous)"/2
  "Power (3ph, Instantaneous)"/2 -> Gain5/1
  "Power (3ph, Instantaneous)"/1 -> Gain/1
  Mux2/1 -> [PQ]
  out/1 -> Demux/1
  Demux/3 -> [Ipcc]
  Demux/2 -> [Vline]
  Demux/1 -> [Iabc]
  Demux/4 -> [Vdc]
  Constant14/1 -> Mux8/2
  Constant13/1 -> Mux12/2
  Mux8/1 -> Sum4/2
  Discrete-Time Integrator2/1 -> Add3/2, Gain15/1
  [Iq] -> Mux7/2
  Add2/1 -> Gain17/1
  Gain15/1 -> Add2/3
  Rate Limiter1/1 -> Add2/1
  Add3/1 -> Gain18/1
  [Vq] -> Mux11/2
  [Id] -> Mux7/1
  [Vd] -> Mux11/1
  Sum5/1 -> Product5/1
  [P] -> Add2/2
  Mux10/1 -> Sum4/1
  Product5/1 -> PID Controller4/1
  dq0 to abc1/1 -> Gain16/1
  Constant6/1 -> Gain13/1
  Demux4/3 -> Terminator5/1
  Gain17/1 -> Product6/2
  [RST] -> PID Controller3/2
  abc to dq1/1 -> Demux4/1
  [RST] -> Switch1/2, Discrete-Time Integrator3/2
  Constant16/1 -> Add1/1
  [RST] -> Product5/2
  PID Controller4/1 -> Scope6/1, Sum7/1
  Add1/1 -> PID Controller5/1
  Sum4/1 -> Scope5/1, Sum5/1
  [Id] -> Virtual Impedance6/1
  Virtual Impedance8/1 -> Sum3/2
  Mux7/1 -> Scope6/2, Sum7/2
  Demux4/1 -> Terminator4/1
  Demux4/2 -> Add1/2
  Switch1/1 -> [theta]
  Sum7/1 -> PID Controller3/1
  Discrete-Time Integrator4/1 -> Switch1/3, [theta_VPCC], abc to dq1/2
  Virtual Impedance7/1 -> Sum3/1
  Constant9/1 -> Mux8/1
  [RST] -> Switch2/2
  Add4/1 -> Discrete-Time Integrator4/1
  [Iq] -> Virtual Impedance5/1
  Sum6/1 -> Mux10/1
  [theta] -> dq0 to abc1/2
  [Iq] -> Virtual Impedance7/1
  Product6/1 -> Discrete-Time Integrator2/1
  Virtual Impedance6/1 -> Sum6/2
  Discrete-Time Integrator3/1 -> Switch1/1
  PID Controller3/1 -> Switch2/1
  Gain14/1 -> Add4/2
  [Vpcc] -> Gain12/1
  RST/1 -> [RST]
  Mux12/1 -> dq0 to abc1/1
  Mux6/1 -> Switch2/3, PID Controller3/3
  Virtual Impedance5/1 -> Sum6/1
  [RST] -> Product6/1
  Gain12/1 -> abc to dq1/1
  Sum3/1 -> Mux10/2
  Gain13/1 -> Add4/1
  [Vd] -> Mux6/1
  Mux11/1 -> Sum5/2, Scope5/2
  Gain18/1 -> Discrete-Time Integrator3/1, [omga]
  [Id] -> Virtual Impedance8/1
  Constant5/1 -> Mux6/2
  Switch2/1 -> Mux12/1
  PID Controller5/1 -> Scope7/1, Gain14/1
  [theta_VPCC] -> Discrete-Time Integrator3/3
  Constant15/1 -> Add3/1
  Constant17/1 -> Switch3/1
  Constant18/1 -> Switch3/3
  [RST] -> Switch3/2
  Switch3/1 -> Rate Limiter1/1
  Bus Creator/1 -> measure/1
  [Ipcc] -> Bus Creator/2
  [omga] -> Bus Creator/4
  [PQ] -> Bus Creator/3
  [Vpcc] -> Bus Creator/1

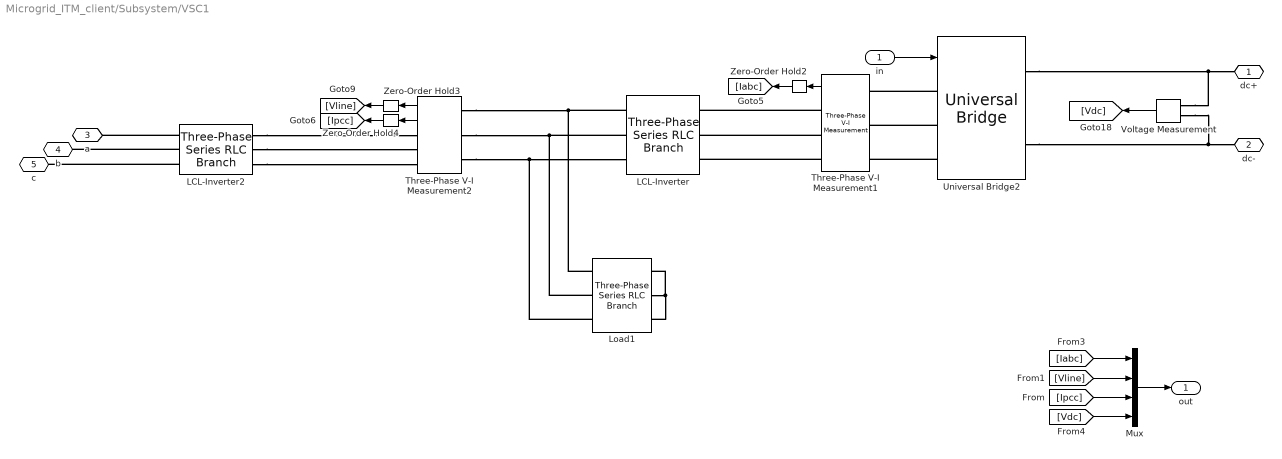
== system Microgrid_ITM_client/Subsystem/VSC1 ==
  in : Inport
  LCL-Inverter : spsThreePhaseSeriesRLCBranchLib/Three-Phase Series RLC Branch  LConnTagsString=A|B|C  RConnTagsString=A|B|C  BranchType=RL  Resistance=0.1  Inductance=Lc  Capacitance=1e-6  Measurements=None
  LCL-Inverter2 : spsThreePhaseSeriesRLCBranchLib/Three-Phase Series RLC Branch  LConnTagsString=A|B|C  RConnTagsString=A|B|C  BranchType=RL  Resistance=0.1  Inductance=0.85e-3  Capacitance=1e-6  Measurements=None
  Load1 : spsThreePhaseSeriesRLCBranchLib/Three-Phase Series RLC Branch  LConnTagsString=A|B|C  RConnTagsString=A|B|C  BranchType=RC  Resistance=0.1  Inductance=1e-3  Capacitance=20e-6  Measurements=None
  Mux : Mux
  Three-Phase V-I Measurement1 : spsThreePhaseVIMeasurementLib/Three-Phase V-I Measurement  VoltageMeasurement=no  SetLabelV=off  LabelV=Vabc  Vpu=off  VpuLL=off  CurrentMeasurement=yes  SetLabelI=off  LabelI=Iabc  Ipu=off  Pbase=100e6  Vbase=500e3  OutputType=Complex  PhasorSimulation=off  PSBequivalent=0
  Three-Phase V-I Measurement2 : spsThreePhaseVIMeasurementLib/Three-Phase V-I Measurement  VoltageMeasurement=phase-to-phase  SetLabelV=off  LabelV=Vabc  Vpu=off  VpuLL=off  CurrentMeasurement=yes  SetLabelI=off  LabelI=Iabc  Ipu=off  Pbase=100e6  Vbase=500e3  OutputType=Complex  PhasorSimulation=off  PSBequivalent=0
  Universal Bridge2 : spsUniversalBridgeLib/Universal Bridge  Arms=3  SnubberResistance=1e5  SnubberCapacitance=inf  Device=IGBT / Diodes  Ron=0.1  Lon=0  ForwardVoltages="[  0  0  ]"  ForwardVoltage=0  GTOparameters=[ 10e-6 , 20e-6 ]  IGBTparameters=[ 1e-6 , 2e-6 ]  Measurements=None  Measurements_2=None  converterType=Rectifier
  Voltage Measurement : spsVoltageMeasurementLib/Voltage Measurement  PhasorSimulation=off  OutputType=Complex  PSBequivalent=0
  Zero-Order Hold2 : ZeroOrderHold  SampleTime=1/fsw1
  Zero-Order Hold3 : ZeroOrderHold  SampleTime=1/fsw1
  Zero-Order Hold4 : ZeroOrderHold  SampleTime=1/fsw1
  dc+ : PMIOPort  Side=Left
  dc- : PMIOPort  Port=2  Side=Left
  a : PMIOPort  Port=3  Side=Right
  b : PMIOPort  Port=4  Side=Right
  c : PMIOPort  Port=5  Side=Right
  out : Outport
  wires:
  Three-Phase V-I Measurement2/2 -> Zero-Order Hold4/1
  Zero-Order Hold4/1 -> [Ipcc]
  Zero-Order Hold3/1 -> [Vline]
  Three-Phase V-I Measurement1/1 -> Zero-Order Hold2/1
  in/1 -> Universal Bridge2/1
  Zero-Order Hold2/1 -> [Iabc]
  Three-Phase V-I Measurement2/1 -> Zero-Order Hold3/1
  [Vdc] -> Mux/4
  [Ipcc] -> Mux/3
  [Vline] -> Mux/2
  [Iabc] -> Mux/1
  Mux/1 -> out/1
  Voltage Measurement/1 -> [Vdc]
  connections:
  Load1/RConn2 -- Load1/RConn3 -- Load1/RConn1
  LCL-Inverter/RConn2 -- Three-Phase V-I Measurement2/LConn2 -- Load1/LConn2
  LCL-Inverter/RConn1 -- Load1/LConn1 -- Three-Phase V-I Measurement2/LConn1
  Three-Phase V-I Measurement2/LConn3 -- LCL-Inverter/RConn3 -- Load1/LConn3
  LCL-Inverter2/LConn2 -- Three-Phase V-I Measurement2/RConn2
  Universal Bridge2/LConn3 -- Three-Phase V-I Measurement1/LConn3
  Three-Phase V-I Measurement1/RConn1 -- LCL-Inverter/LConn1
  LCL-Inverter2/RConn1 -- a/RConn1
  LCL-Inverter2/LConn1 -- Three-Phase V-I Measurement2/RConn1
  LCL-Inverter2/RConn2 -- b/RConn1
  Three-Phase V-I Measurement1/RConn2 -- LCL-Inverter/LConn2
  LCL-Inverter2/LConn3 -- Three-Phase V-I Measurement2/RConn3
  LCL-Inverter2/RConn3 -- c/RConn1
  Universal Bridge2/LConn1 -- Three-Phase V-I Measurement1/LConn1
  Universal Bridge2/LConn2 -- Three-Phase V-I Measurement1/LConn2
  Three-Phase V-I Measurement1/RConn3 -- LCL-Inverter/LConn3
  Universal Bridge2/RConn1 -- dc+/RConn1 -- Voltage Measurement/LConn1
  Universal Bridge2/RConn2 -- dc-/RConn1 -- Voltage Measurement/LConn2

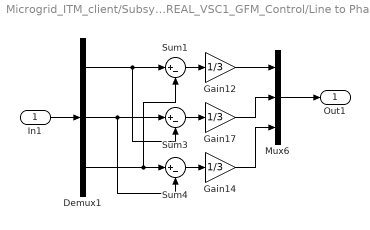
== system Microgrid_ITM_client/Subsystem/REAL_VSC1_GFM_Control/Line to Phase ==
  In1 : Inport
  Demux1 : Demux  Outputs=3
  Gain12 : Gain  Gain=1/3
  Gain14 : Gain  Gain=1/3
  Gain17 : Gain  Gain=1/3
  Mux6 : Mux  Inputs=3
  Sum1 : Sum  Inputs=|+-
  Sum3 : Sum  Inputs=|+-
  Sum4 : Sum  Inputs=|+-
  Out1 : Outport
  wires:
  Demux1/1 -> Sum1/1, Sum3/2
  Mux6/1 -> Out1/1
  Gain12/1 -> Mux6/1
  Demux1/2 -> Sum3/1, Sum4/2
  Demux1/3 -> Sum1/2, Sum4/1
  Sum4/1 -> Gain14/1
  Sum1/1 -> Gain12/1
  Gain14/1 -> Mux6/3
  In1/1 -> Demux1/1
  Gain17/1 -> Mux6/2
  Sum3/1 -> Gain17/1
